simulink model "MotorModel"  (R2022a)
settings: Solver=ode4  StartTime=0.0  StopTime=30  FixedStep=0.001  RelTol=1e-3
libraries: dspsrcs4 x2
settings Model: Creator=randolf  LastModifiedBy=randolf

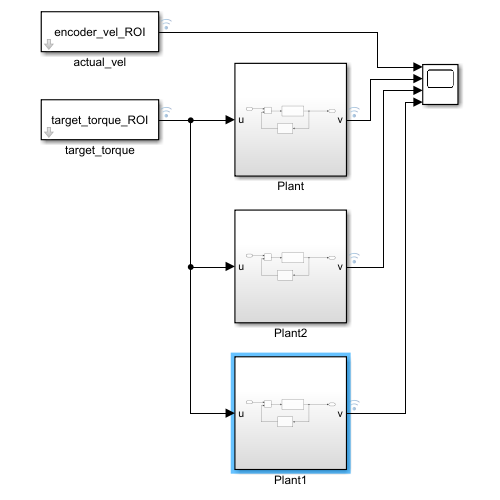
[thumbnail: Simulink's stored preview of the top-level diagram]
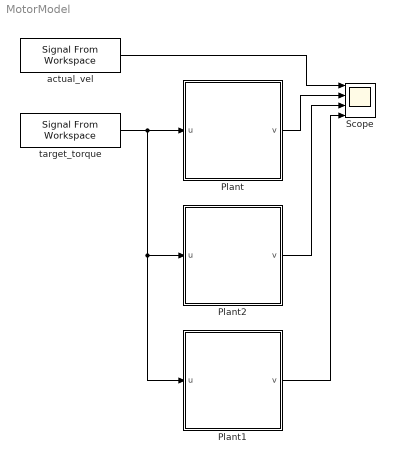
== system MotorModel ==
  Plant : Subsystem
  Plant1 : Subsystem
  Plant2 : Subsystem
  Scope : Scope  NumInputPorts=4
  actual_vel : dspsrcs4/Signal From Workspace  X=encoder_vel_ROI  Ts=0.001  nsamps=1  OutputAfterFinalValue=Setting to zero  ignoreOrWarnInputAndFrameLengths=off  OutputFrames=off
  target_torque : dspsrcs4/Signal From Workspace  X=target_torque_ROI  Ts=0.001  nsamps=1  OutputAfterFinalValue=Setting to zero  ignoreOrWarnInputAndFrameLengths=off  OutputFrames=off
  wires:
  target_torque/1 -> Plant1/1(u), Plant2/1(u), Plant/1(u)
  actual_vel/1 -> Scope/1
  Plant/1(v) -> Scope/2
  Plant2/1(v) -> Scope/3
  Plant1/1(v) -> Scope/4

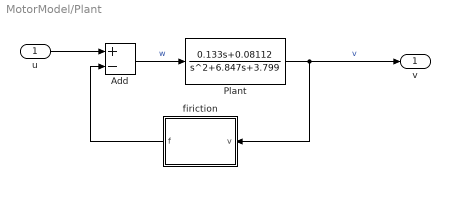
== system MotorModel/Plant ==
  u : Inport
  Add : Sum  Inputs=+-
  Plant : TransferFcn  Numerator=[0.133 0.08112]  Denominator=[1 6.847 3.799]
  firiction : MATLAB Function  TreatAsAtomicUnit=on
  v : Outport
  wires:
  Add/1 -> Plant/1  "w"
  u/1 -> Add/1
  Plant/1 -> v/1, firiction/1(v)  "v"
  firiction/1(f) -> Add/2

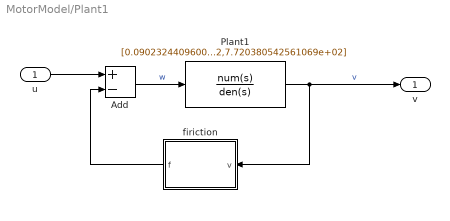
== system MotorModel/Plant1 ==
  u : Inport
  Add : Sum  Inputs=+-
  Plant1 : TransferFcn  Numerator=[0.090232440960097,3.051715207136733,19.382986592459790]  Denominator=[1,20.527749511328590,2.672042521178649e+02,7.720380542561069e+02]
  firiction : MATLAB Function  TreatAsAtomicUnit=on
  v : Outport
  wires:
  Add/1 -> Plant1/1  "w"
  u/1 -> Add/1
  Plant1/1 -> v/1, firiction/1(v)  "v"
  firiction/1(f) -> Add/2

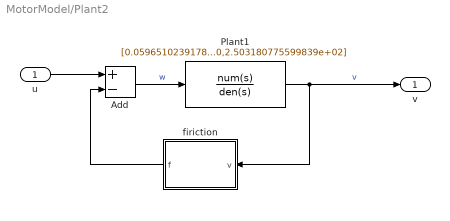
== system MotorModel/Plant2 ==
  u : Inport
  Add : Sum  Inputs=+-
  Plant1 : TransferFcn  Numerator=[0.059651023917809,5.389055599068365]  Denominator=[1,33.166974989873530,2.503180775599839e+02]
  firiction : MATLAB Function  TreatAsAtomicUnit=on
  v : Outport
  wires:
  firiction/1(f) -> Add/2
  Plant1/1 -> firiction/1(v), v/1  "v"
  u/1 -> Add/1
  Add/1 -> Plant1/1  "w"

== matlab function MotorModel/Plant/firiction ==
  data: v input; f output
function f = fcn(v)
    if (v>0)
        f = 135.5;
    else
        f = -136.7;
    end
end

== matlab function MotorModel/Plant1/firiction ==
  data: v input; f output
function f = fcn(v)
    if (v>0)
        f = 153;
    else
        f = -154;
    end
end

== matlab function MotorModel/Plant2/firiction ==
  data: v input; f output
function f = fcn(v)
    if (v>0)
        f = 135.5;
    else
        f = -136.7;
    end
end
